simulink model "sampleModel1_pp_1_1"  (R2021b)
settings: Solver=VariableStepAuto  StartTime=0.0  StopTime=10.0  RelTol=1e-3
undefined symbols (not defined in the file or in its folder): DiscIntNeverNeededParam, Newton, Raphson
libraries: simulink x18, slpidlib x4
settings Model: Creator=user  LastModifiedBy=cemery

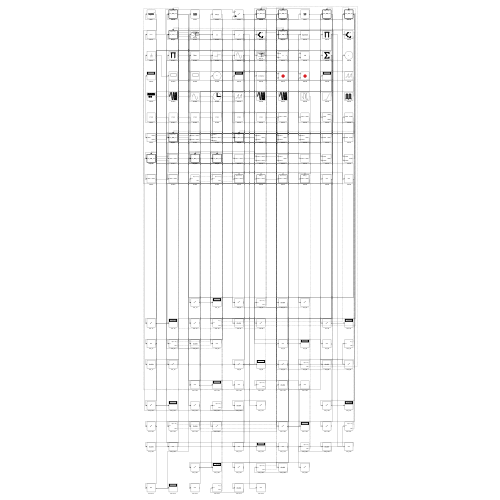
[thumbnail: Simulink's stored preview of the top-level diagram]
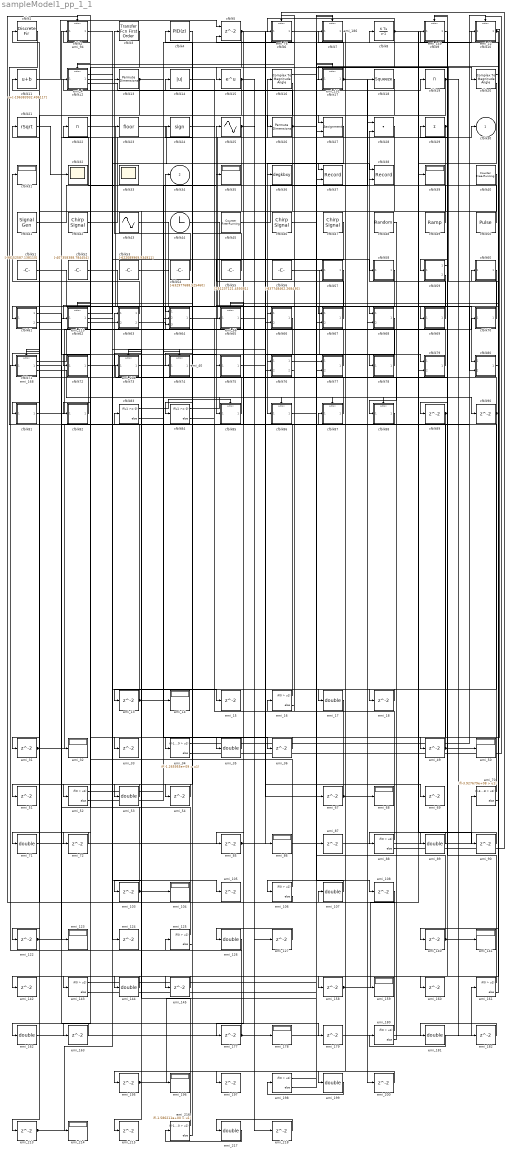
== system sampleModel1_pp_1_1 ==
  cfblk1 : DiscreteFir  SampleTime=1
  cfblk10 : Subsystem  TreatAsAtomicUnit=on
  cfblk11 : Bias  Bias=[-196383932.496117]
  cfblk12 : Subsystem  TreatAsAtomicUnit=on
  cfblk13 : PermuteDimensions
  cfblk14 : Abs
  cfblk15 : Math  SaturateOnIntegerOverflow=on
  cfblk16 : ComplexToMagnitudeAngle
  cfblk17 : Subsystem  TreatAsAtomicUnit=on
  cfblk18 : Squeeze
  cfblk19 : Product  Inputs=*
  cfblk2 : Subsystem  TreatAsAtomicUnit=on
  cfblk20 : ComplexToMagnitudeAngle
  cfblk21 : Sqrt  Operator=rSqrt  AlgorithmType=Newton-Raphson  SaturateOnIntegerOverflow=on
  cfblk22 : Product  Inputs=*
  cfblk23 : Rounding
  cfblk24 : Signum
  cfblk25 : Sin  TimeSource=Use external signal  SampleTime=0
  cfblk26 : PermuteDimensions
  cfblk27 : Assignment  DiagnosticForDimensions=Warning  IndexOptions=Index vector (dialog)  Indices=1  OutputSizes=1
  cfblk28 : DotProduct  InputSameDT=on  OutDataTypeStr=Inherit: Inherit via internal rule
  cfblk29 : Sum  Inputs=+
  cfblk3 : simulink/Discrete/Transfer Fcn First Order  PoleZ=0.95  ICPrevOutput=0.0  DoSatur=off
  cfblk31 : Display
  cfblk32 : Scope
  cfblk33 : Scope
      settings: Floating=on
  cfblk35 : Display
  cfblk36 : ToWorkspace  VariableName=degkbxy  SaveFormat=Timeseries  SampleTime=-1
  cfblk37 : Record  FileSettingsInternal="{\"entries\":[{\"content\":{\"excelSettings\":{\"content\":{},\"type\":\"Streamout.ExcelSettings\"}},\"type\":\"Streamout.FileSettingStorage\",\"uuid\":\"f10d7984-3c8e-4a01-b437-64e6950a7f1c\"}],\"packageUris\":[\"http://schema.mathworks.com/mf0/streamout_blocks/R2020a\"],\"version\":\"1.0\"}"  Layout=[1 1]  SignalsInternal="{\"entries\":[{\"content\":{\"signals\":[{\"content\":{\"blockPath\":[\"sampleModel1_pp_1_1/cfblk37\"],\"channel\":[],\"dimensions\":[1],\"domain\":\"sampleModel1_pp_1_1/cfblk37\",\"lineColor\":\"#77ac30\",\"plots\":[],\"port\":1,\"sid\":[\"\"],\"signalID\":978,\"signalName\":\"cfblk14\"},\"type\":\"RecordBlkView.Signal\",\"uuid\":\"64c2965d-c8c3-42f9-aeb4-1a9e7a6147a8\"},{\"content\":{\"blockPath\":[\"sampleModel1_pp_1_1/cfblk37\"],\"channel\":[],\"dimensions\":[1],\"domain\":\"sampleModel1_pp_1_1/cfblk37\",\"lineColor\":\"#4dbeee\",\"plots\":[],\"port\":2,\"sid\":[\"\"],\"signalID\":982,\"signalName\":\"cfblk16:1\"},\"type\":\"RecordBlkView.Signal\",\"uuid\":\"42395b9b-3004-4283-a0bf-fe2a9eef8989\"}]},\"type\":\"RecordBlkView.InputSignals\",\"uuid\":\"5b0a9ef9-d487-431f-a20f-830121fcf74f\"}],\"packageUris\":[\"http://schema.mathworks.com/mf0/streamout_blocks/R2020a\"],\"version\":\"1.0\"}"  VisualizationBindings="{\"xyplotplugin\":{\"info\":[{\"series\":[],\"subplotID\":1}]}}"  CompatibilityTag=XY
  cfblk38 : Record  FileSettingsInternal="{\"entries\":[{\"content\":{\"excelSettings\":{\"content\":{},\"type\":\"Streamout.ExcelSettings\"}},\"type\":\"Streamout.FileSettingStorage\",\"uuid\":\"de5ebdad-7bfa-474c-9602-9eb7a528d104\"}],\"packageUris\":[\"http://schema.mathworks.com/mf0/streamout_blocks/R2020a\"],\"version\":\"1.0\"}"  Layout=[1 1]  SignalsInternal="{\"entries\":[{\"content\":{\"signals\":[{\"content\":{\"blockPath\":[\"sampleModel1_pp_1_1/cfblk38\"],\"channel\":[],\"dimensions\":[1],\"domain\":\"sampleModel1_pp_1_1/cfblk38\",\"lineColor\":\"#a2142f\",\"plots\":[],\"port\":1,\"sid\":[\"\"],\"signalID\":986,\"signalName\":\"cfblk2\"},\"type\":\"RecordBlkView.Signal\",\"uuid\":\"59823cac-66f4-4fb3-a1c8-ec7d4885dc8b\"},{\"content\":{\"blockPath\":[\"sampleModel1_pp_1_1/cfblk38\"],\"channel\":[],\"dimensions\":[1],\"domain\":\"sampleModel1_pp_1_1/cfblk38\",\"lineColor\":\"#139fff\",\"plots\":[],\"port\":2,\"sid\":[\"\"],\"signalID\":990,\"signalName\":\"cfblk49\"},\"type\":\"RecordBlkView.Signal\",\"uuid\":\"f4fb396b-3304-46b4-a061-728441c3573f\"}]},\"type\":\"RecordBlkView.InputSignals\",\"uuid\":\"8e89f174-1f5e-4363-8739-2fa17bc2ac55\"}],\"packageUris\":[\"http://schema.mathworks.com/mf0/streamout_blocks/R2020a\"],\"version\":\"1.0\"}"  VisualizationBindings="{\"xyplotplugin\":{\"info\":[{\"series\":[],\"subplotID\":1}]}}"  CompatibilityTag=XY
  cfblk39 : Display
  cfblk4 : slpidlib/PID Controller  Controller=PID  Form=Parallel  TimeDomain=Discrete-time  UseExternalTs=off  SampleTime=1  IntegratorMethod=Forward Euler  FilterMethod=Forward Euler  ControllerParametersSource=internal  P=1  I=1  D=0  UseFilter=on  N=100  TunerSelectOption=Transfer Function Based (PID Tuner App)  InitialConditionSource=internal  InitialConditionForIntegrator=0  InitialConditionForFilter=0  DifferentiatorICPrevScaledInput=0  ExternalReset=none  TrackingMode=off  Kt=1  LimitOutput=off  SatLimitsSource=internal  UpperSaturationLimit=inf  LowerSaturationLimit=-inf  LinearizeAsGain=off  AntiWindupMode=none  Kb=1  POutMin=[]  POutMax=[]  IOutMin=[]  IOutMax=[]  DOutMin=[]  DOutMax=[]  NOutMin=[]  NOutMax=[]  SumOutMin=[]  SumOutMax=[]  SaturationOutMin=[]  SaturationOutMax=[]  PParamMin=[]  PParamMax=[]  IParamMin=[]  IParamMax=[]  DParamMin=[]  DParamMax=[]  NParamMin=[]  NParamMax=[]  KbParamMin=[]  KbParamMax=[]  KtParamMin=[]  KtParamMax=[]  KbOutMin=[]  KbOutMax=[]  KtOutMin=[]  KtOutMax=[]  IntegratorOutMin=[]  IntegratorOutMax=[]  FilterOutMin=[]  FilterOutMax=[]  SumI1OutMin=[]  SumI1OutMax=[]  SumI2OutMin=[]  SumI2OutMax=[]  SumI3OutMin=[]  SumI3OutMax=[]  SumI4OutMin=[]  SumI4OutMax=[]  SumDOutMin=[]  SumDOutMax=[]  DifferentiatorOutMin=[]  DifferentiatorOutMax=[]  FilterDiffOutCoefMin=[]  FilterDiffOutCoefMax=[]  ReciprocalOutMin=[]  ReciprocalOutMax=[]  SumDenOutMin=[]  SumDenOutMax=[]  SumNumOutMin=[]  SumNumOutMax=[]  DivideOutMin=[]  DivideOutMax=[]  UdiffTsProdOutMin=[]  UdiffTsProdOutMax=[]  NTsProdOutMin=[]  NTsProdOutMax=[]  UintegralTsProdOutMin=[]  UintegralTsProdOutMax=[]  UngainTsProdOutMin=[]  UngainTsProdOutMax=[]  IntegratorContinuousStateAttributes=''  IntegratorStateMustResolveToSignalObject=off  IntegratorRTWStateStorageClass=Auto  FilterContinuousStateAttributes=''  FilterStateMustResolveToSignalObject=off  FilterRTWStateStorageClass=Auto  ParallelPVariant=InternalParameters  IdealPVariant=Disabled  IVariant=InternalParameters  DVariant=InternalParameters  IntegratorVariant=Discrete  SatVariant=Disabled  AWVariant=Passthrough  PCopyVariant=Disabled  TRVariant=Disabled  FdbkBlocksVariant=Forward  IdealPFdbkVariant=Disabled  SatFdbkVariant=Disabled  DerivativeFilterVariant=ForwardEulerFilter  NVariant=InternalParameters  NCopyVariant=Disabled  FilterICVariant=InternalICsFilter  IntegratorICVariant=InternalICs  ExternalResetVariant=Disabled  TRSumVariant=Passthrough  SumFdbkVariant=Disabled  SumVariant=Sum_PID  TsampFilterVariant=InternalTs  TsampNgainVariant=Passthrough  TsampIntegralVariant=Passthrough  ExternalSaturationOutDataTypeStr=Inherit: Same as second input
  cfblk40 : simulink/Sources/Counter Free-Running  NumBits=[29.000000]  tsamp=-1
  cfblk41 : SignalGenerator  WaveForm=square  Amplitude=[-21494723.199962]
  cfblk42 : simulink/Sources/Chirp Signal  f1=[-261506437.759570]  T=[-777594489.412425]  f2=[560504136.642276]
  cfblk43 : Sin  Amplitude=[-220522326.077493]  Bias=[-516617428.172335]  SampleTime=0
  cfblk44 : Clock
  cfblk45 : simulink/Sources/Counter Free-Running  NumBits=[24.000000]  tsamp=-1
  cfblk46 : simulink/Sources/Chirp Signal  f1=[-807090949.663223]  T=[-736053414.787330]  f2=[884101181.550970]
  cfblk47 : simulink/Sources/Chirp Signal  f1=[912269080.459605]  T=[150417190.156931]  f2=[-880440914.105688]
  cfblk48 : RandomNumber  Mean=[-53044.017326]  Variance=[35315.857122]  Seed=[821194040.000000]  SampleTime=0.1
  cfblk49 : simulink/Sources/Ramp  slope=[-9691.931247]  start=[3.108166]  InitialOutput=[-662019.941075]
  cfblk5 : Delay  ShowEnablePort=on  SampleTime=1
      settings: InputPortMap=u0,e6
  cfblk50 : DiscretePulseGenerator  PulseType=Time based  Amplitude=[298230949.912904]  Period=[73172238.834145]  PulseWidth=5  PhaseDelay=[6.000000]
  cfblk51 : Constant  Value=[-98152587.138110]  SampleTime=1
  cfblk52 : Constant  Value=[-407358388.784454]  SampleTime=1
  cfblk53 : Constant  Value=[-622089969.934911]  SampleTime=1
  cfblk54 : Constant  Value=[-632977688.525460]  SampleTime=1
  cfblk55 : Constant  Value=[251237121.459381]  SampleTime=1
  cfblk56 : Constant  Value=[-837748462.268430]  SampleTime=1
  cfblk57 : Subsystem
  cfblk58 : Subsystem
  cfblk59 : Subsystem
  cfblk6 : Subsystem  TreatAsAtomicUnit=on
  cfblk60 : Subsystem
  cfblk61 : Subsystem
  cfblk62 : Subsystem  TreatAsAtomicUnit=on
  cfblk63 : Subsystem
  cfblk64 : Subsystem
  cfblk65 : Subsystem  TreatAsAtomicUnit=on
  cfblk66 : Subsystem
  cfblk67 : Subsystem
  cfblk68 : Subsystem
  cfblk69 : Subsystem
  cfblk7 : Subsystem  TreatAsAtomicUnit=on
  cfblk70 : Subsystem
  cfblk71 : Subsystem  TreatAsAtomicUnit=on
  cfblk72 : Subsystem
  cfblk73 : Subsystem  TreatAsAtomicUnit=on
  cfblk74 : Subsystem  TreatAsAtomicUnit=on
  cfblk75 : Subsystem
  cfblk76 : Subsystem
  cfblk77 : Subsystem
  cfblk78 : Subsystem
  cfblk79 : Subsystem
  cfblk8 : DiscreteIntegrator  ICPrevOutput=DiscIntNeverNeededParam  ICPrevScaledInput=DiscIntNeverNeededParam
  cfblk80 : Subsystem
  cfblk81 : Subsystem
  cfblk82 : Subsystem
  cfblk83 : If  IfExpression=u1 >= 0  SampleTime=1
  cfblk84 : If  IfExpression=u1 >= 0  SampleTime=1
  cfblk85 : Subsystem  TreatAsAtomicUnit=on
  cfblk86 : Subsystem  TreatAsAtomicUnit=on
  cfblk87 : Subsystem  TreatAsAtomicUnit=on
  cfblk88 : Subsystem  TreatAsAtomicUnit=on
  cfblk89 : Delay  SampleTime=1
  cfblk9 : Subsystem  TreatAsAtomicUnit=on
  cfblk90 : Delay  SampleTime=1
  emi_{13,15,31,33,67,69,85,87,103,105,140,142,158,160,195,197} (16 alike) : Delay
  emi_{14,32,50,68,86,104,123,141,159,178,196,214} (12 alike) : Display
  emi_{16,52,88,106,125,143,161,180,198} (9 alike) : If  IfExpression=0 > u1
  emi_{17,35,53,71,89,107,126,144,162,181,199,217} (12 alike) : DataTypeConversion  OutDataTypeStr=double
  emi_{18,90,108,127,163,182} (6 alike) : Delay  InitialCondition=0
  emi_113 : Subsystem  TreatAsAtomicUnit=on
  emi_{49,51,122,124,177,179,213,215} (8 alike) : Delay  SampleTime=1
  emi_131 : Subsystem  TreatAsAtomicUnit=on
  emi_145 : Delay  InitialCondition=0.026958
  emi_149 : Subsystem  TreatAsAtomicUnit=on
  emi_168 : Subsystem  TreatAsAtomicUnit=on
  emi_186 : Subsystem  TreatAsAtomicUnit=on
  emi_200 : Delay  InitialCondition=0.16419
  emi_204 : Subsystem  TreatAsAtomicUnit=on
  emi_216 : If  IfExpression=-1.586211e+00 > u1
  emi_218 : Delay  InitialCondition=-0.79311
  emi_22 : Subsystem  TreatAsAtomicUnit=on
  emi_34 : If  IfExpression=-1.265955e+09 > u1
  emi_36 : Delay  InitialCondition=-632977688.5255
  emi_4 : Subsystem  TreatAsAtomicUnit=on
  emi_40 : Subsystem  TreatAsAtomicUnit=on
  emi_54 : Delay  InitialCondition=711045611.6918
  emi_58 : Subsystem  TreatAsAtomicUnit=on
  emi_70 : If  IfExpression=-3.927679e+08 > u1
  emi_72 : Delay  InitialCondition=-196383937.6215
  emi_76 : Subsystem  TreatAsAtomicUnit=on
  emi_94 : Subsystem  TreatAsAtomicUnit=on
  cfblk30 : Outport
  cfblk34 : Outport  Port=2
  wires:
  cfblk63/1(cfblk2) -> cfblk31/1
  cfblk67/1(cfblk2) -> cfblk25/1
  cfblk44/1 -> cfblk68/1(cfblk1)
  cfblk21/1 -> cfblk32/1
  cfblk79/1(cfblk2) -> cfblk34/1
  cfblk69/1(cfblk2) -> cfblk28/2
  cfblk72/1(cfblk2) -> cfblk29/1
  cfblk70/1(cfblk2) -> cfblk15/1
  cfblk23/1 -> cfblk86/1(cfblk1)
  cfblk43/1 -> cfblk66/1(cfblk1)
  cfblk77/1(cfblk2) -> cfblk11/1
  cfblk48/1 -> cfblk88/1(cfblk1)
  cfblk53/1 -> cfblk80/1(cfblk1)
  cfblk64/1(cfblk2) -> cfblk30/1
  cfblk68/1(cfblk2) -> cfblk76/1(cfblk1)
  cfblk50/1 -> cfblk22/1
  cfblk78/1(cfblk2) -> cfblk4/1
  cfblk85/1(cfblk2) -> cfblk63/1(cfblk1)
  cfblk52/1 -> cfblk69/1(cfblk1)
  cfblk76/1(cfblk2) -> cfblk77/1(cfblk1)
  cfblk1/1 -> cfblk87/1(cfblk1)
  cfblk56/1 -> cfblk79/1(cfblk1)
  cfblk47/1 -> cfblk85/1(cfblk1)
  cfblk45/1 -> cfblk18/1
  cfblk51/1 -> cfblk80/2(cfblk3)
  cfblk59/2(cfblk3) -> cfblk63/2(cfblk4)
  cfblk81/1(cfblk2) -> cfblk70/1(cfblk1)
  cfblk66/1(cfblk2) -> cfblk84/1
  cfblk86/1(cfblk2) -> cfblk57/1(cfblk1)
  cfblk75/1(cfblk2) -> cfblk8/1
  cfblk42/1 -> cfblk16/1
  cfblk4/1 -> cfblk64/1(cfblk1)
  cfblk22/1 -> cfblk64/2(cfblk3)
  cfblk41/1 -> cfblk3/1
  cfblk20/1 -> cfblk67/1(cfblk1)
  cfblk58/1(cfblk2) -> cfblk61/1(cfblk1)
  cfblk49/1 -> cfblk38/2
  cfblk14/1 -> cfblk37/1
  cfblk80/1(cfblk2) -> cfblk60/1(cfblk1)
  cfblk20/2 -> cfblk79/2(cfblk3)
  cfblk54/1 -> cfblk13/1
  cfblk28/1 -> cfblk68/2(cfblk5)
  cfblk87/1(cfblk2) -> cfblk21/1
  cfblk11/1 -> cfblk5/1
  cfblk57/1(cfblk2) -> cfblk67/2(cfblk4)
  cfblk82/1(cfblk2) -> cfblk1/1
  cfblk61/1(cfblk2) -> cfblk75/1(cfblk1)
  cfblk88/1(cfblk2) -> cfblk83/1
  cfblk60/1(cfblk2) -> cfblk81/1(cfblk1)
  cfblk16/1 -> cfblk37/2
  cfblk76/2(cfblk5) -> cfblk5/2
  cfblk18/1 -> cfblk27/2
  cfblk27/1 -> cfblk36/1
  cfblk3/1 -> cfblk72/1(cfblk1)
  cfblk46/1 -> cfblk77/2(cfblk4)
  cfblk16/2 -> cfblk26/1
  cfblk61/2(cfblk3) -> cfblk23/1
  cfblk63/2(cfblk5) -> cfblk64/3(cfblk4)
  cfblk55/1 -> cfblk24/1
  cfblk40/1 -> cfblk82/1(cfblk1)
  cfblk24/1 -> cfblk66/2(cfblk5)
  cfblk83/1 -> cfblk85/Action
  cfblk83/2 -> cfblk86/Action
  cfblk84/1 -> cfblk87/Action
  cfblk84/2 -> cfblk88/Action
  cfblk59/1(cfblk2) -> cfblk89/1
  cfblk90/1 -> cfblk12/1(emi_1), emi_13/1, emi_18/1
  cfblk12/1(emi_2) -> cfblk58/1(cfblk1)
  cfblk12/2(emi_3) -> cfblk19/1
  emi_13/1 -> emi_4/1(emi_11), emi_14/1
  emi_4/1(emi_12) -> emi_15/1
  emi_16/2 -> cfblk12/Action
  emi_16/1 -> emi_4/Action
  emi_17/1 -> emi_16/1
  emi_18/1 -> emi_17/1
  cfblk13/1 -> cfblk10/1(emi_20), emi_31/1, emi_36/1
  emi_31/1 -> emi_22/1(emi_29), emi_32/1
  emi_22/1(emi_30) -> emi_33/1
  emi_34/2 -> cfblk10/Action
  emi_34/1 -> emi_22/Action
  emi_35/1 -> emi_34/1
  emi_36/1 -> emi_35/1
  cfblk29/1 -> cfblk74/1(emi_38), emi_49/1, emi_54/1
  cfblk74/1(emi_39) -> cfblk14/1
  emi_49/1 -> emi_40/1(emi_47), emi_50/1
  emi_40/1(emi_48) -> emi_51/1
  emi_52/2 -> cfblk74/Action
  emi_52/1 -> emi_40/Action
  emi_53/1 -> emi_52/1
  emi_54/1 -> emi_53/1
  cfblk5/1 -> cfblk65/1(emi_56), emi_67/1, emi_72/1
  cfblk65/1(emi_57) -> cfblk78/1(cfblk1)
  emi_67/1 -> emi_58/1(emi_65), emi_68/1
  emi_58/1(emi_66) -> emi_69/1
  emi_70/2 -> cfblk65/Action
  emi_70/1 -> emi_58/Action
  emi_71/1 -> emi_70/1
  emi_72/1 -> emi_71/1
  cfblk8/1 -> cfblk6/1(emi_74), emi_85/1, emi_90/1
  cfblk6/1(emi_75) -> cfblk20/1
  emi_85/1 -> emi_76/1(emi_83), emi_86/1
  emi_76/1(emi_84) -> emi_87/1
  emi_88/2 -> cfblk6/Action
  emi_88/1 -> emi_76/Action
  emi_89/1 -> emi_88/1
  emi_90/1 -> emi_89/1
  cfblk26/1 -> cfblk2/1(emi_92), emi_103/1, emi_108/1
  cfblk2/1(emi_93) -> cfblk38/1
  emi_103/1 -> emi_94/1(emi_101), emi_104/1
  emi_94/1(emi_102) -> emi_105/1
  emi_106/2 -> cfblk2/Action
  emi_106/1 -> emi_94/Action
  emi_107/1 -> emi_106/1
  emi_108/1 -> emi_107/1
  cfblk15/1 -> cfblk62/1(emi_110), emi_122/1, emi_127/1
  cfblk62/1(emi_111) -> cfblk28/1
  cfblk62/2(emi_112) -> cfblk76/2(cfblk4)
  emi_122/1 -> emi_113/1(emi_120), emi_123/1
  emi_113/1(emi_121) -> emi_124/1
  emi_125/2 -> cfblk62/Action
  emi_125/1 -> emi_113/Action
  emi_126/1 -> emi_125/1
  emi_127/1 -> emi_126/1
  cfblk10/1(emi_21) -> cfblk17/1(emi_129), emi_140/1, emi_145/1
  emi_140/1 -> emi_131/1(emi_138), emi_141/1
  emi_131/1(emi_139) -> emi_142/1
  emi_143/2 -> cfblk17/Action
  emi_143/1 -> emi_131/Action
  emi_144/1 -> emi_143/1
  emi_145/1 -> emi_144/1
  cfblk89/1 -> cfblk9/1(emi_147), emi_158/1, emi_163/1
  cfblk9/1(emi_148) -> cfblk59/1(cfblk1)
  emi_158/1 -> emi_149/1(emi_156), emi_159/1
  emi_149/1(emi_157) -> emi_160/1
  emi_161/2 -> cfblk9/Action
  emi_161/1 -> emi_149/Action
  emi_162/1 -> emi_161/1
  emi_163/1 -> emi_162/1
  cfblk19/1 -> cfblk71/1(emi_165), emi_177/1, emi_182/1
  cfblk71/1(emi_166) -> cfblk39/1
  cfblk71/2(emi_167) -> cfblk90/1
  emi_177/1 -> emi_168/1(emi_175), emi_178/1
  emi_168/1(emi_176) -> emi_179/1
  emi_180/2 -> cfblk71/Action
  emi_180/1 -> emi_168/Action
  emi_181/1 -> emi_180/1
  emi_182/1 -> emi_181/1
  cfblk17/1(emi_130) -> cfblk7/1(emi_184), emi_195/1, emi_200/1
  cfblk7/1(emi_185) -> cfblk27/1
  emi_195/1 -> emi_186/1(emi_193), emi_196/1
  emi_186/1(emi_194) -> emi_197/1
  emi_198/2 -> cfblk7/Action
  emi_198/1 -> emi_186/Action
  emi_199/1 -> emi_198/1
  emi_200/1 -> emi_199/1
  cfblk25/1 -> cfblk73/1(emi_202), emi_213/1, emi_218/1
  cfblk73/1(emi_203) -> cfblk35/1
  emi_213/1 -> emi_204/1(emi_211), emi_214/1
  emi_204/1(emi_212) -> emi_215/1
  emi_216/2 -> cfblk73/Action
  emi_216/1 -> emi_204/Action
  emi_217/1 -> emi_216/1
  emi_218/1 -> emi_217/1

== system sampleModel1_pp_1_1/cfblk10 ==
  emi_20 : Inport
  Action Port : ActionPort  ActionPortLabel=else
  cfblk10 : Trigonometry
  emi_21 : Outport
  wires:
  emi_20/1 -> cfblk10/1
  cfblk10/1 -> emi_21/1

== system sampleModel1_pp_1_1/cfblk12 ==
  emi_1 : Inport
  Action Port : ActionPort  ActionPortLabel=else
  cfblk12 : ComplexToMagnitudeAngle
  emi_2 : Outport
  emi_3 : Outport  Port=2
  wires:
  emi_1/1 -> cfblk12/1
  cfblk12/1 -> emi_2/1
  cfblk12/2 -> emi_3/1

== system sampleModel1_pp_1_1/cfblk17 ==
  emi_129 : Inport
  Action Port : ActionPort  ActionPortLabel=else
  cfblk17 : Sqrt  SaturateOnIntegerOverflow=on
  emi_130 : Outport
  wires:
  emi_129/1 -> cfblk17/1
  cfblk17/1 -> emi_130/1

== system sampleModel1_pp_1_1/cfblk2 ==
  emi_92 : Inport
  Action Port : ActionPort  ActionPortLabel=else
  cfblk2 : simulink/Discrete/Transfer Fcn First Order  PoleZ=0.95  ICPrevOutput=0.0  DoSatur=off
  emi_93 : Outport
  wires:
  emi_92/1 -> cfblk2/1
  cfblk2/1 -> emi_93/1

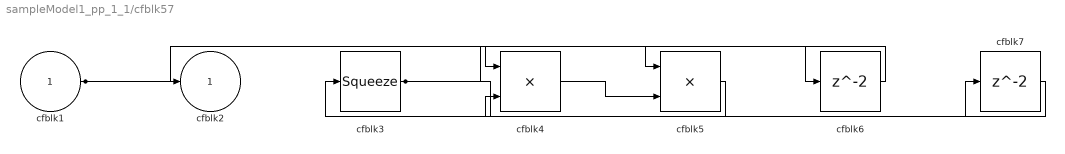
== system sampleModel1_pp_1_1/cfblk57 ==
  cfblk1 : Inport
  cfblk3 : Squeeze
  cfblk4 : Product
  cfblk5 : Product
  cfblk6 : Delay  SampleTime=1
  cfblk7 : Delay  SampleTime=1
  cfblk2 : Outport
  wires:
  cfblk3/1 -> cfblk6/1, cfblk7/1
  cfblk5/1 -> cfblk3/1
  cfblk1/1 -> cfblk4/1, cfblk2/1
  cfblk4/1 -> cfblk5/2
  cfblk6/1 -> cfblk5/1
  cfblk7/1 -> cfblk4/2

== system sampleModel1_pp_1_1/cfblk58 ==
  cfblk1 : Inport
  cfblk3 : DotProduct  InputSameDT=on  OutDataTypeStr=Inherit: Inherit via internal rule
  cfblk2 : Outport
  wires:
  cfblk1/1 -> cfblk3/1, cfblk3/2
  cfblk3/1 -> cfblk2/1

== system sampleModel1_pp_1_1/cfblk59 ==
  cfblk1 : Inport
  cfblk2 : Outport
  cfblk3 : Outport  Port=2
  wires:
  cfblk1/1 -> cfblk2/1, cfblk3/1

== system sampleModel1_pp_1_1/cfblk6 ==
  emi_74 : Inport
  Action Port : ActionPort  ActionPortLabel=else
  cfblk6 : simulink/Discrete/Difference  ICPrevInput=0.0  OutMin=[]  OutMax=[]  OutDataTypeStr=Inherit: Inherit via back propagation  OutDataType=fixdt(1, 16)  OutScaling=2^-10  DoSatur=off
  emi_75 : Outport
  wires:
  emi_74/1 -> cfblk6/1
  cfblk6/1 -> emi_75/1

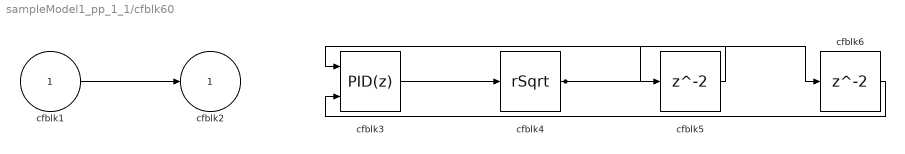
== system sampleModel1_pp_1_1/cfblk60 ==
  cfblk1 : Inport
  cfblk3 : slpidlib/PID Controller (2DOF)  Controller=PID  Form=Parallel  TimeDomain=Discrete-time  UseExternalTs=off  SampleTime=1  IntegratorMethod=Forward Euler  FilterMethod=Forward Euler  ControllerParametersSource=internal  P=1  I=1  D=0  UseFilter=on  N=100  b=1  c=1  TunerSelectOption=Transfer Function Based (PID Tuner App)  InitialConditionSource=internal  InitialConditionForIntegrator=0  InitialConditionForFilter=0  DifferentiatorICPrevScaledInput=0  ExternalReset=none  TrackingMode=off  Kt=1  LimitOutput=off  SatLimitsSource=internal  UpperSaturationLimit=inf  LowerSaturationLimit=-inf  LinearizeAsGain=off  AntiWindupMode=none  Kb=1  POutMin=[]  POutMax=[]  IOutMin=[]  IOutMax=[]  DOutMin=[]  DOutMax=[]  NOutMin=[]  NOutMax=[]  bOutMin=[]  bOutMax=[]  cOutMin=[]  cOutMax=[]  SumOutMin=[]  SumOutMax=[]  SaturationOutMin=[]  SaturationOutMax=[]  PParamMin=[]  PParamMax=[]  IParamMin=[]  IParamMax=[]  DParamMin=[]  DParamMax=[]  NParamMin=[]  NParamMax=[]  bParamMin=[]  bParamMax=[]  cParamMin=[]  cParamMax=[]  KbParamMin=[]  KbParamMax=[]  KtParamMin=[]  KtParamMax=[]  KbOutMin=[]  KbOutMax=[]  KtOutMin=[]  KtOutMax=[]  IntegratorOutMin=[]  IntegratorOutMax=[]  FilterOutMin=[]  FilterOutMax=[]  SumI1OutMin=[]  SumI1OutMax=[]  SumI2OutMin=[]  SumI2OutMax=[]  SumI3OutMin=[]  SumI3OutMax=[]  SumI4OutMin=[]  SumI4OutMax=[]  SumDOutMin=[]  SumDOutMax=[]  Sum1OutMin=[]  Sum1OutMax=[]  Sum2OutMin=[]  Sum2OutMax=[]  Sum3OutMin=[]  Sum3OutMax=[]  DifferentiatorOutMin=[]  DifferentiatorOutMax=[]  FilterDiffOutCoefMin=[]  FilterDiffOutCoefMax=[]  ReciprocalOutMin=[]  ReciprocalOutMax=[]  SumDenOutMin=[]  SumDenOutMax=[]  SumNumOutMin=[]  SumNumOutMax=[]  DivideOutMin=[]  DivideOutMax=[]  UdiffTsProdOutMin=[]  UdiffTsProdOutMax=[]  NTsProdOutMin=[]  NTsProdOutMax=[]  UintegralTsProdOutMin=[]  UintegralTsProdOutMax=[]  UngainTsProdOutMin=[]  UngainTsProdOutMax=[]  IntegratorContinuousStateAttributes=''  IntegratorStateMustResolveToSignalObject=off  IntegratorRTWStateStorageClass=Auto  FilterContinuousStateAttributes=''  FilterStateMustResolveToSignalObject=off  FilterRTWStateStorageClass=Auto  ParallelPVariant=InternalParameters  IdealPVariant=Disabled  IVariant=InternalParameters  DVariant=InternalParameters  bVariant=InternalParameters  cVariant=InternalParameters  IntegratorVariant=Discrete  SatVariant=Disabled  AWVariant=Passthrough  PCopyVariant=Disabled  TRVariant=Disabled  FdbkBlocksVariant=Forward  IdealPFdbkVariant=Disabled  SatFdbkVariant=Disabled  DerivativeFilterVariant=ForwardEulerFilter  NVariant=InternalParameters  NCopyVariant=Disabled  FilterICVariant=InternalICsFilter  IntegratorICVariant=InternalICs  ExternalResetVariant=Disabled  TRSumVariant=Passthrough  SumFdbkVariant=Disabled  SumVariant=Sum_PID  TsampFilterVariant=InternalTs  TsampNgainVariant=Passthrough  TsampIntegralVariant=Passthrough  ExternalSaturationOutDataTypeStr=Inherit: Same as second input
      settings: SourceProductBaseCode=SL
  cfblk4 : Sqrt  Operator=rSqrt  AlgorithmType=Newton-Raphson  SaturateOnIntegerOverflow=on
  cfblk5 : Delay  SampleTime=1
  cfblk6 : Delay  SampleTime=1
  cfblk2 : Outport
  wires:
  cfblk4/1 -> cfblk5/1, cfblk6/1
  cfblk1/1 -> cfblk2/1
  cfblk3/1 -> cfblk4/1
  cfblk5/1 -> cfblk3/1
  cfblk6/1 -> cfblk3/2

== system sampleModel1_pp_1_1/cfblk61 ==
  cfblk1 : Inport
  cfblk2 : Outport
  cfblk3 : Outport  Port=2
  wires:
  cfblk1/1 -> cfblk3/1, cfblk2/1

== system sampleModel1_pp_1_1/cfblk62 ==
  emi_110 : Inport
  Action Port : ActionPort  ActionPortLabel=else
  cfblk62 : Subsystem
  emi_111 : Outport
  emi_112 : Outport  Port=2
  wires:
  emi_110/1 -> cfblk62/1(cfblk1)
  cfblk62/1(cfblk2) -> emi_111/1
  cfblk62/2(cfblk4) -> emi_112/1

== system sampleModel1_pp_1_1/cfblk63 ==
  cfblk1 : Inport
  cfblk4 : Inport  Port=2
  cfblk3 : DiscreteFir  SampleTime=1
  cfblk2 : Outport
  cfblk5 : Outport  Port=2
  wires:
  cfblk4/1 -> cfblk3/1
  cfblk3/1 -> cfblk2/1
  cfblk1/1 -> cfblk5/1

== system sampleModel1_pp_1_1/cfblk64 ==
  cfblk1 : Inport
  cfblk3 : Inport  Port=2
  cfblk4 : Inport  Port=3
  cfblk2 : Outport
  wires:
  cfblk4/1 -> cfblk2/1

== system sampleModel1_pp_1_1/cfblk65 ==
  emi_56 : Inport
  Action Port : ActionPort  ActionPortLabel=else
  cfblk65 : Subsystem
  emi_57 : Outport
  wires:
  emi_56/1 -> cfblk65/1(cfblk1)
  cfblk65/1(cfblk2) -> emi_57/1

== system sampleModel1_pp_1_1/cfblk66 ==
  cfblk1 : Inport
  cfblk5 : Inport  Port=2
  cfblk3 : simulink/Discrete/Transfer Fcn Real Zero  ZeroZ=0.75  ICPrevInput=0.0  DoSatur=off
      settings: SourceProductBaseCode=SL
  cfblk4 : Sum
  cfblk2 : Outport
  wires:
  cfblk5/1 -> cfblk4/1
  cfblk1/1 -> cfblk3/1
  cfblk4/1 -> cfblk2/1
  cfblk3/1 -> cfblk4/2

== system sampleModel1_pp_1_1/cfblk67 ==
  cfblk1 : Inport
  cfblk4 : Inport  Port=2
  cfblk3 : simulink/Discrete/Transfer Fcn Lead or Lag  PoleZ=0.95  ZeroZ=0.75  ICPrevOutput=0.0  ICPrevInput=0.0  DoSatur=off
      settings: SourceProductBaseCode=SL
  cfblk2 : Outport
  wires:
  cfblk1/1 -> cfblk3/1
  cfblk4/1 -> cfblk2/1

== system sampleModel1_pp_1_1/cfblk68 ==
  cfblk1 : Inport
  cfblk5 : Inport  Port=2
  cfblk3 : simulink/Math Operations/MinMax Running Resettable  Function=min  vinit=0.0
  cfblk4 : Constant  Value=[650627590.804091]  SampleTime=1
  cfblk2 : Outport
  wires:
  cfblk1/1 -> cfblk2/1
  cfblk5/1 -> cfblk3/1
  cfblk4/1 -> cfblk3/2

== system sampleModel1_pp_1_1/cfblk69 ==
  cfblk1 : Inport
  cfblk3 : Rounding
  cfblk4 : Reshape
  cfblk2 : Outport
  wires:
  cfblk3/1 -> cfblk2/1
  cfblk4/1 -> cfblk3/1
  cfblk1/1 -> cfblk4/1

== system sampleModel1_pp_1_1/cfblk7 ==
  emi_184 : Inport
  Action Port : ActionPort  ActionPortLabel=else
  cfblk7 : simulink/Discrete/Difference  ICPrevInput=0.0  OutMin=[]  OutMax=[]  OutDataTypeStr=Inherit: Inherit via back propagation  OutDataType=fixdt(1, 16)  OutScaling=2^-10  DoSatur=off
  emi_185 : Outport
  wires:
  emi_184/1 -> cfblk7/1
  cfblk7/1 -> emi_185/1

== system sampleModel1_pp_1_1/cfblk70 ==
  cfblk1 : Inport
  cfblk3 : DiscreteFilter  SampleTime=1
  cfblk4 : UnaryMinus
  cfblk2 : Outport
  wires:
  cfblk1/1 -> cfblk4/1
  cfblk4/1 -> cfblk3/1
  cfblk3/1 -> cfblk2/1

== system sampleModel1_pp_1_1/cfblk71 ==
  emi_165 : Inport
  Action Port : ActionPort  ActionPortLabel=else
  cfblk71 : Subsystem
  emi_166 : Outport
  emi_167 : Outport  Port=2
  wires:
  emi_165/1 -> cfblk71/1(cfblk1)
  cfblk71/1(cfblk2) -> emi_166/1
  cfblk71/2(cfblk5) -> emi_167/1

== system sampleModel1_pp_1_1/cfblk72 ==
  cfblk1 : Inport
  cfblk3 : DiscreteStateSpace
  cfblk4 : ComplexToMagnitudeAngle
  cfblk5 : Constant  Value=[711045611.691823]  SampleTime=1
  cfblk2 : Outport
  wires:
  cfblk1/1 -> cfblk3/1
  cfblk4/1 -> cfblk2/1
  cfblk5/1 -> cfblk4/1

== system sampleModel1_pp_1_1/cfblk73 ==
  emi_202 : Inport
  Action Port : ActionPort  ActionPortLabel=else
  cfblk73 : Subsystem
  emi_203 : Outport
  wires:
  emi_202/1 -> cfblk73/1(cfblk1)
  cfblk73/1(cfblk2) -> emi_203/1

== system sampleModel1_pp_1_1/cfblk74 ==
  emi_38 : Inport
  Action Port : ActionPort  ActionPortLabel=else
  cfblk74 : Subsystem
  emi_39 : Outport
  wires:
  emi_38/1 -> cfblk74/1(cfblk1)
  cfblk74/1(cfblk2) -> emi_39/1

== system sampleModel1_pp_1_1/cfblk75 ==
  cfblk1 : Inport
  cfblk3 : DiscreteStateSpace
  cfblk4 : Reshape
  cfblk5 : Delay  SampleTime=1
  cfblk2 : Outport
  wires:
  cfblk1/1 -> cfblk2/1
  cfblk3/1 -> cfblk4/1
  cfblk4/1 -> cfblk5/1
  cfblk5/1 -> cfblk3/1

== system sampleModel1_pp_1_1/cfblk76 ==
  cfblk1 : Inport
  cfblk4 : Inport  Port=2
  cfblk3 : Assignment  DiagnosticForDimensions=Warning  IndexOptions=Index vector (dialog)  Indices=1  OutputSizes=1
  cfblk2 : Outport
  cfblk5 : Outport  Port=2
  wires:
  cfblk4/1 -> cfblk3/1
  cfblk1/1 -> cfblk3/2
  cfblk3/1 -> cfblk2/1, cfblk5/1

== system sampleModel1_pp_1_1/cfblk77 ==
  cfblk1 : Inport
  cfblk4 : Inport  Port=2
  cfblk3 : Product
  cfblk2 : Outport
  wires:
  cfblk4/1 -> cfblk3/1
  cfblk1/1 -> cfblk3/2
  cfblk3/1 -> cfblk2/1

== system sampleModel1_pp_1_1/cfblk78 ==
  cfblk1 : Inport
  cfblk3 : simulink/Discrete/Transfer Fcn Lead or Lag  PoleZ=0.95  ZeroZ=0.75  ICPrevOutput=0.0  ICPrevInput=0.0  DoSatur=off
      settings: SourceProductBaseCode=SL
  cfblk4 : Math  Operator=mod  SaturateOnIntegerOverflow=on
  cfblk5 : Constant  Value=[350664131.493999]  SampleTime=1
  cfblk2 : Outport
  wires:
  cfblk4/1 -> cfblk3/1
  cfblk1/1 -> cfblk4/1
  cfblk3/1 -> cfblk2/1
  cfblk5/1 -> cfblk4/2

== system sampleModel1_pp_1_1/cfblk79 ==
  cfblk1 : Inport
  cfblk3 : Inport  Port=2
  cfblk2 : Outport
  wires:
  cfblk1/1 -> cfblk2/1

== system sampleModel1_pp_1_1/cfblk80 ==
  cfblk1 : Inport
  cfblk3 : Inport  Port=2
  cfblk2 : Outport
  wires:
  cfblk1/1 -> cfblk2/1

== system sampleModel1_pp_1_1/cfblk81 ==
  cfblk1 : Inport
  cfblk3 : simulink/Discrete/Tapped Delay  vinit=0.0  samptime=-1  NumDelays=1  DelayOrder=Oldest  includeCurrent=off
  cfblk4 : DotProduct  InputSameDT=on  OutDataTypeStr=Inherit: Inherit via internal rule
  cfblk2 : Outport
  wires:
  cfblk4/1 -> cfblk2/1
  cfblk1/1 -> cfblk3/1
  cfblk3/1 -> cfblk4/1, cfblk4/2

== system sampleModel1_pp_1_1/cfblk82 ==
  cfblk1 : Inport
  cfblk3 : Constant  Value=[358033508.186404]  SampleTime=1
  cfblk4 : Constant  Value=[890348226.218803]  SampleTime=1
  cfblk2 : Outport
  wires:
  cfblk1/1 -> cfblk2/1

== system sampleModel1_pp_1_1/cfblk85 ==
  cfblk1 : Inport
  Action Port : ActionPort  ActionPortLabel=if(u1 >= 0)
  cfblk3 : simulink/Math Operations/Slider Gain  gain=1  low=0  high=2
  cfblk4 : Constant  Value=[-299563973.117790]  SampleTime=1
  cfblk2 : Outport
  wires:
  cfblk4/1 -> cfblk2/1
  cfblk1/1 -> cfblk3/1

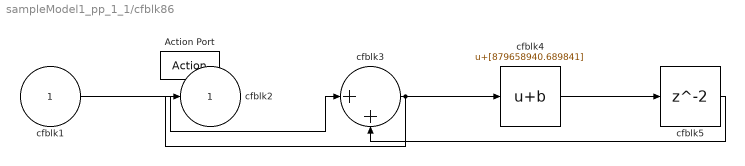
== system sampleModel1_pp_1_1/cfblk86 ==
  cfblk1 : Inport
  Action Port : ActionPort  ActionPortLabel=else
  cfblk3 : Sum  Inputs=|++
  cfblk4 : Bias  Bias=[879658940.689841]
  cfblk5 : Delay
  cfblk2 : Outport
  wires:
  cfblk1/1 -> cfblk3/1
  cfblk3/1 -> cfblk4/1, cfblk2/1
  cfblk4/1 -> cfblk5/1
  cfblk5/1 -> cfblk3/2

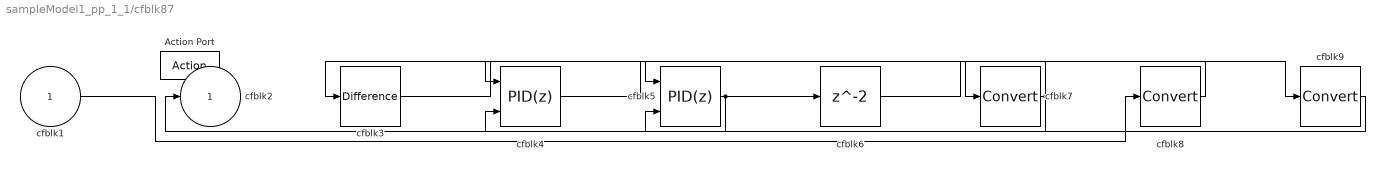
== system sampleModel1_pp_1_1/cfblk87 ==
  cfblk1 : Inport
  Action Port : ActionPort  ActionPortLabel=if(u1 >= 0)
  cfblk3 : simulink/Discrete/Difference  ICPrevInput=0.0  OutMin=[]  OutMax=[]  OutDataTypeStr=Inherit: Inherit via back propagation  OutDataType=fixdt(1, 16)  OutScaling=2^-10  DoSatur=off
  cfblk4 : slpidlib/PID Controller (2DOF)  Controller=PID  Form=Parallel  TimeDomain=Discrete-time  UseExternalTs=off  SampleTime=-1  IntegratorMethod=Forward Euler  FilterMethod=Forward Euler  ControllerParametersSource=internal  P=1  I=1  D=0  UseFilter=on  N=100  b=1  c=1  TunerSelectOption=Transfer Function Based (PID Tuner App)  InitialConditionSource=internal  InitialConditionForIntegrator=0  InitialConditionForFilter=0  DifferentiatorICPrevScaledInput=0  ExternalReset=none  TrackingMode=off  Kt=1  LimitOutput=off  SatLimitsSource=internal  UpperSaturationLimit=inf  LowerSaturationLimit=-inf  LinearizeAsGain=off  AntiWindupMode=none  Kb=1  POutMin=[]  POutMax=[]  IOutMin=[]  IOutMax=[]  DOutMin=[]  DOutMax=[]  NOutMin=[]  NOutMax=[]  bOutMin=[]  bOutMax=[]  cOutMin=[]  cOutMax=[]  SumOutMin=[]  SumOutMax=[]  SaturationOutMin=[]  SaturationOutMax=[]  PParamMin=[]  PParamMax=[]  IParamMin=[]  IParamMax=[]  DParamMin=[]  DParamMax=[]  NParamMin=[]  NParamMax=[]  bParamMin=[]  bParamMax=[]  cParamMin=[]  cParamMax=[]  KbParamMin=[]  KbParamMax=[]  KtParamMin=[]  KtParamMax=[]  KbOutMin=[]  KbOutMax=[]  KtOutMin=[]  KtOutMax=[]  IntegratorOutMin=[]  IntegratorOutMax=[]  FilterOutMin=[]  FilterOutMax=[]  SumI1OutMin=[]  SumI1OutMax=[]  SumI2OutMin=[]  SumI2OutMax=[]  SumI3OutMin=[]  SumI3OutMax=[]  SumI4OutMin=[]  SumI4OutMax=[]  SumDOutMin=[]  SumDOutMax=[]  Sum1OutMin=[]  Sum1OutMax=[]  Sum2OutMin=[]  Sum2OutMax=[]  Sum3OutMin=[]  Sum3OutMax=[]  DifferentiatorOutMin=[]  DifferentiatorOutMax=[]  FilterDiffOutCoefMin=[]  FilterDiffOutCoefMax=[]  ReciprocalOutMin=[]  ReciprocalOutMax=[]  SumDenOutMin=[]  SumDenOutMax=[]  SumNumOutMin=[]  SumNumOutMax=[]  DivideOutMin=[]  DivideOutMax=[]  UdiffTsProdOutMin=[]  UdiffTsProdOutMax=[]  NTsProdOutMin=[]  NTsProdOutMax=[]  UintegralTsProdOutMin=[]  UintegralTsProdOutMax=[]  UngainTsProdOutMin=[]  UngainTsProdOutMax=[]  IntegratorContinuousStateAttributes=''  IntegratorStateMustResolveToSignalObject=off  IntegratorRTWStateStorageClass=Auto  FilterContinuousStateAttributes=''  FilterStateMustResolveToSignalObject=off  FilterRTWStateStorageClass=Auto  ParallelPVariant=InternalParameters  IdealPVariant=Disabled  IVariant=InternalParameters  DVariant=InternalParameters  bVariant=InternalParameters  cVariant=InternalParameters  IntegratorVariant=Discrete  SatVariant=Disabled  AWVariant=Passthrough  PCopyVariant=Disabled  TRVariant=Disabled  FdbkBlocksVariant=Forward  IdealPFdbkVariant=Disabled  SatFdbkVariant=Disabled  DerivativeFilterVariant=ForwardEulerFilter  NVariant=InternalParameters  NCopyVariant=Disabled  FilterICVariant=InternalICsFilter  IntegratorICVariant=InternalICs  ExternalResetVariant=Disabled  TRSumVariant=Passthrough  SumFdbkVariant=Disabled  SumVariant=Sum_PID  TsampFilterVariant=InternalTs  TsampNgainVariant=Passthrough  TsampIntegralVariant=Passthrough  ExternalSaturationOutDataTypeStr=Inherit: Same as second input
      settings: SourceProductBaseCode=SL
  cfblk5 : slpidlib/PID Controller (2DOF)  Controller=PID  Form=Parallel  TimeDomain=Discrete-time  UseExternalTs=off  SampleTime=-1  IntegratorMethod=Forward Euler  FilterMethod=Forward Euler  ControllerParametersSource=internal  P=1  I=1  D=0  UseFilter=on  N=100  b=1  c=1  TunerSelectOption=Transfer Function Based (PID Tuner App)  InitialConditionSource=internal  InitialConditionForIntegrator=0  InitialConditionForFilter=0  DifferentiatorICPrevScaledInput=0  ExternalReset=none  TrackingMode=off  Kt=1  LimitOutput=off  SatLimitsSource=internal  UpperSaturationLimit=inf  LowerSaturationLimit=-inf  LinearizeAsGain=off  AntiWindupMode=none  Kb=1  POutMin=[]  POutMax=[]  IOutMin=[]  IOutMax=[]  DOutMin=[]  DOutMax=[]  NOutMin=[]  NOutMax=[]  bOutMin=[]  bOutMax=[]  cOutMin=[]  cOutMax=[]  SumOutMin=[]  SumOutMax=[]  SaturationOutMin=[]  SaturationOutMax=[]  PParamMin=[]  PParamMax=[]  IParamMin=[]  IParamMax=[]  DParamMin=[]  DParamMax=[]  NParamMin=[]  NParamMax=[]  bParamMin=[]  bParamMax=[]  cParamMin=[]  cParamMax=[]  KbParamMin=[]  KbParamMax=[]  KtParamMin=[]  KtParamMax=[]  KbOutMin=[]  KbOutMax=[]  KtOutMin=[]  KtOutMax=[]  IntegratorOutMin=[]  IntegratorOutMax=[]  FilterOutMin=[]  FilterOutMax=[]  SumI1OutMin=[]  SumI1OutMax=[]  SumI2OutMin=[]  SumI2OutMax=[]  SumI3OutMin=[]  SumI3OutMax=[]  SumI4OutMin=[]  SumI4OutMax=[]  SumDOutMin=[]  SumDOutMax=[]  Sum1OutMin=[]  Sum1OutMax=[]  Sum2OutMin=[]  Sum2OutMax=[]  Sum3OutMin=[]  Sum3OutMax=[]  DifferentiatorOutMin=[]  DifferentiatorOutMax=[]  FilterDiffOutCoefMin=[]  FilterDiffOutCoefMax=[]  ReciprocalOutMin=[]  ReciprocalOutMax=[]  SumDenOutMin=[]  SumDenOutMax=[]  SumNumOutMin=[]  SumNumOutMax=[]  DivideOutMin=[]  DivideOutMax=[]  UdiffTsProdOutMin=[]  UdiffTsProdOutMax=[]  NTsProdOutMin=[]  NTsProdOutMax=[]  UintegralTsProdOutMin=[]  UintegralTsProdOutMax=[]  UngainTsProdOutMin=[]  UngainTsProdOutMax=[]  IntegratorContinuousStateAttributes=''  IntegratorStateMustResolveToSignalObject=off  IntegratorRTWStateStorageClass=Auto  FilterContinuousStateAttributes=''  FilterStateMustResolveToSignalObject=off  FilterRTWStateStorageClass=Auto  ParallelPVariant=InternalParameters  IdealPVariant=Disabled  IVariant=InternalParameters  DVariant=InternalParameters  bVariant=InternalParameters  cVariant=InternalParameters  IntegratorVariant=Discrete  SatVariant=Disabled  AWVariant=Passthrough  PCopyVariant=Disabled  TRVariant=Disabled  FdbkBlocksVariant=Forward  IdealPFdbkVariant=Disabled  SatFdbkVariant=Disabled  DerivativeFilterVariant=ForwardEulerFilter  NVariant=InternalParameters  NCopyVariant=Disabled  FilterICVariant=InternalICsFilter  IntegratorICVariant=InternalICs  ExternalResetVariant=Disabled  TRSumVariant=Passthrough  SumFdbkVariant=Disabled  SumVariant=Sum_PID  TsampFilterVariant=InternalTs  TsampNgainVariant=Passthrough  TsampIntegralVariant=Passthrough  ExternalSaturationOutDataTypeStr=Inherit: Same as second input
      settings: SourceProductBaseCode=SL
  cfblk6 : Delay
  cfblk7 : DataTypeConversion
  cfblk8 : DataTypeConversion
  cfblk9 : DataTypeConversion
  cfblk2 : Outport
  wires:
  cfblk3/1 -> cfblk5/1
  cfblk4/1 -> cfblk7/1
  cfblk5/1 -> cfblk2/1, cfblk6/1
  cfblk7/1 -> cfblk3/1, cfblk5/2
  cfblk1/1 -> cfblk8/1
  cfblk8/1 -> cfblk4/1
  cfblk6/1 -> cfblk9/1
  cfblk9/1 -> cfblk4/2

== system sampleModel1_pp_1_1/cfblk88 ==
  cfblk1 : Inport
  Action Port : ActionPort  ActionPortLabel=else
  cfblk3 : Sin  TimeSource=Use external signal  SampleTime=0
  cfblk4 : Constant  Value=[40104934.780774]  SampleTime=1
  cfblk2 : Outport
  wires:
  cfblk3/1 -> cfblk2/1
  cfblk1/1 -> cfblk3/1

== system sampleModel1_pp_1_1/cfblk9 ==
  emi_147 : Inport
  Action Port : ActionPort  ActionPortLabel=else
  cfblk9 : simulink/Discrete/Transfer Fcn First Order  PoleZ=0.95  ICPrevOutput=0.0  DoSatur=off
  emi_148 : Outport
  wires:
  emi_147/1 -> cfblk9/1
  cfblk9/1 -> emi_148/1

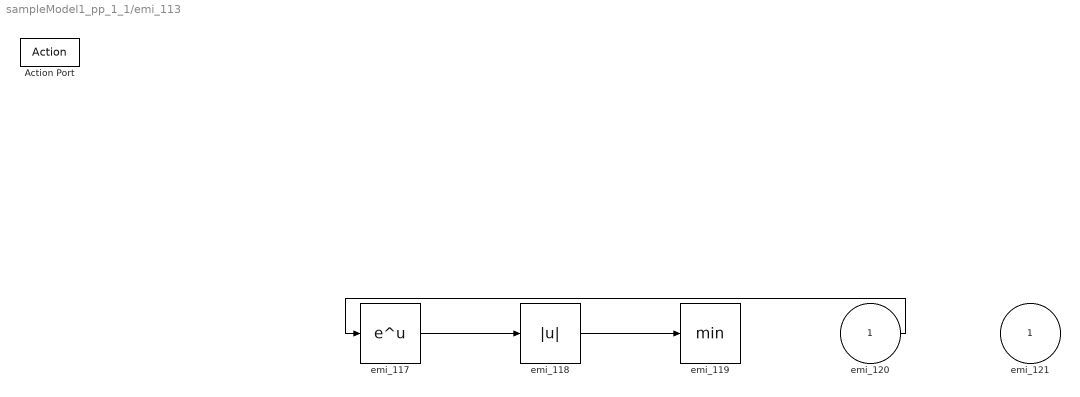
== system sampleModel1_pp_1_1/emi_113 ==
  emi_120 : Inport
  Action Port : ActionPort  ActionPortLabel=if(0 > u1)
  emi_117 : Math  SaturateOnIntegerOverflow=on
  emi_118 : Abs
  emi_119 : MinMax
  emi_121 : Outport
  wires:
  emi_120/1 -> emi_117/1
  emi_117/1 -> emi_118/1
  emi_118/1 -> emi_119/1

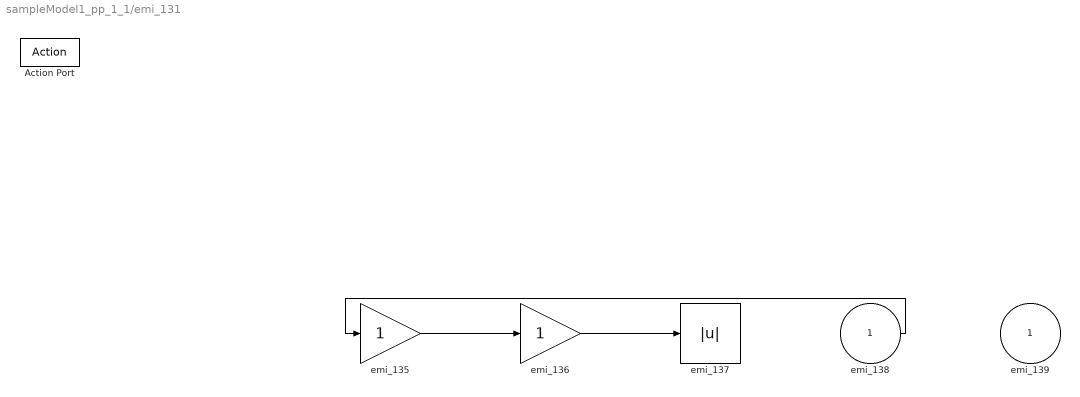
== system sampleModel1_pp_1_1/emi_131 ==
  emi_138 : Inport
  Action Port : ActionPort  ActionPortLabel=if(0 > u1)
  emi_135 : Gain
  emi_136 : Gain
  emi_137 : Abs
  emi_139 : Outport
  wires:
  emi_138/1 -> emi_135/1
  emi_135/1 -> emi_136/1
  emi_136/1 -> emi_137/1

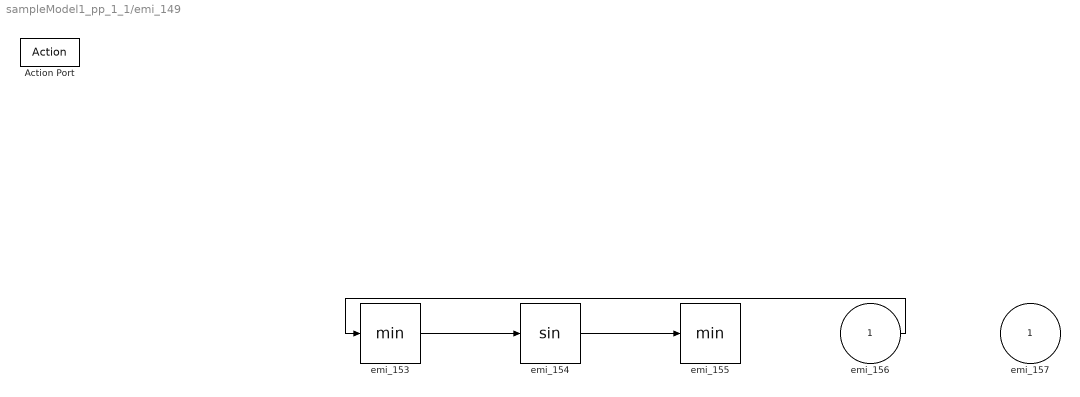
== system sampleModel1_pp_1_1/emi_149 ==
  emi_156 : Inport
  Action Port : ActionPort  ActionPortLabel=if(0 > u1)
  emi_153 : MinMax
  emi_154 : Trigonometry
  emi_155 : MinMax
  emi_157 : Outport
  wires:
  emi_156/1 -> emi_153/1
  emi_153/1 -> emi_154/1
  emi_154/1 -> emi_155/1

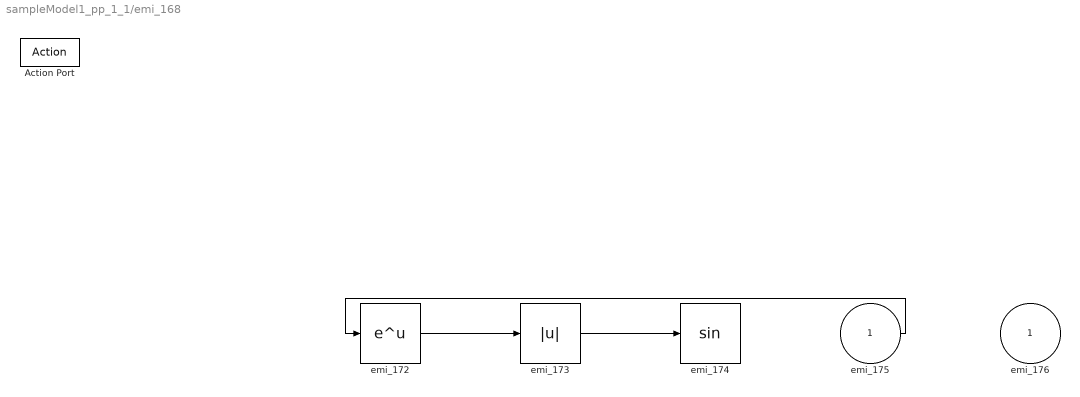
== system sampleModel1_pp_1_1/emi_168 ==
  emi_175 : Inport
  Action Port : ActionPort  ActionPortLabel=if(0 > u1)
  emi_172 : Math  SaturateOnIntegerOverflow=on
  emi_173 : Abs
  emi_174 : Trigonometry
  emi_176 : Outport
  wires:
  emi_175/1 -> emi_172/1
  emi_172/1 -> emi_173/1
  emi_173/1 -> emi_174/1

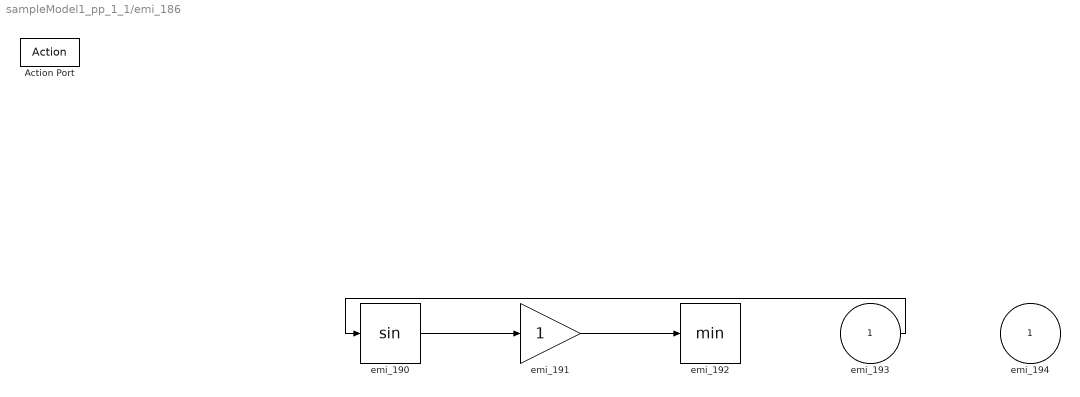
== system sampleModel1_pp_1_1/emi_186 ==
  emi_193 : Inport
  Action Port : ActionPort  ActionPortLabel=if(0 > u1)
  emi_190 : Trigonometry
  emi_191 : Gain
  emi_192 : MinMax
  emi_194 : Outport
  wires:
  emi_193/1 -> emi_190/1
  emi_190/1 -> emi_191/1
  emi_191/1 -> emi_192/1

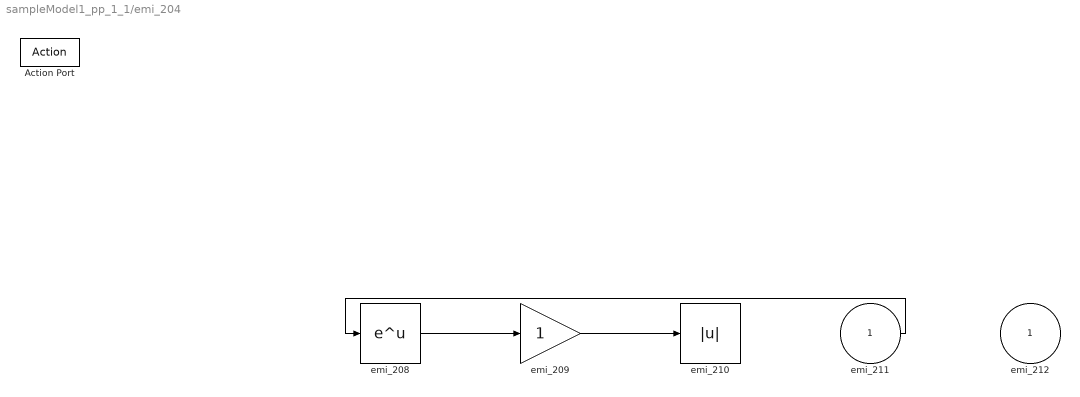
== system sampleModel1_pp_1_1/emi_204 ==
  emi_211 : Inport
  Action Port : ActionPort  ActionPortLabel=if(-1.586211e+00 > u1)
  emi_208 : Math  SaturateOnIntegerOverflow=on
  emi_209 : Gain
  emi_210 : Abs
  emi_212 : Outport
  wires:
  emi_211/1 -> emi_208/1
  emi_208/1 -> emi_209/1
  emi_209/1 -> emi_210/1

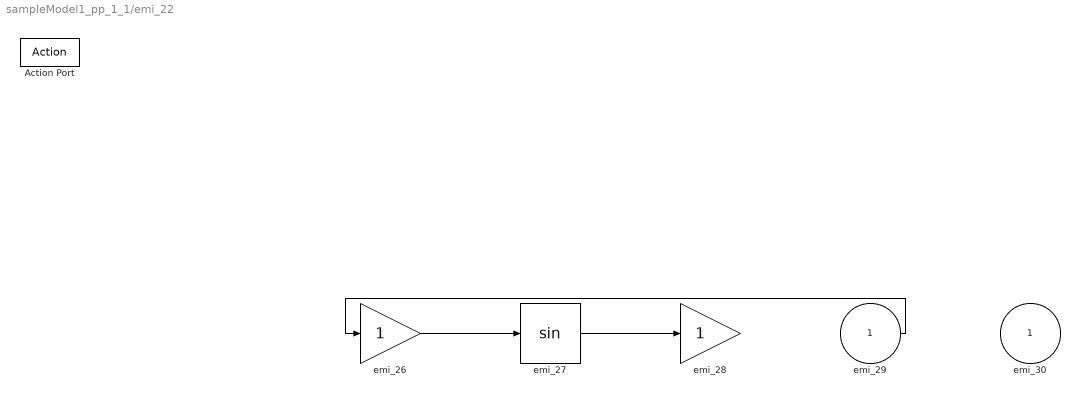
== system sampleModel1_pp_1_1/emi_22 ==
  emi_29 : Inport
  Action Port : ActionPort  ActionPortLabel=if(-1.265955e+09 > u1)
  emi_26 : Gain
  emi_27 : Trigonometry
  emi_28 : Gain
  emi_30 : Outport
  wires:
  emi_29/1 -> emi_26/1
  emi_26/1 -> emi_27/1
  emi_27/1 -> emi_28/1

== system sampleModel1_pp_1_1/emi_4 ==
  emi_11 : Inport
  Action Port : ActionPort  ActionPortLabel=if(0 > u1)
  emi_10 : Math  SaturateOnIntegerOverflow=on
  emi_8 : Trigonometry
  emi_9 : Math  SaturateOnIntegerOverflow=on
  emi_12 : Outport
  wires:
  emi_11/1 -> emi_8/1
  emi_8/1 -> emi_9/1
  emi_9/1 -> emi_10/1

== system sampleModel1_pp_1_1/emi_40 ==
  emi_47 : Inport
  Action Port : ActionPort  ActionPortLabel=if(0 > u1)
  emi_44 : MinMax
  emi_45 : Trigonometry
  emi_46 : Gain
  emi_48 : Outport
  wires:
  emi_47/1 -> emi_44/1
  emi_44/1 -> emi_45/1
  emi_45/1 -> emi_46/1

== system sampleModel1_pp_1_1/emi_58 ==
  emi_65 : Inport
  Action Port : ActionPort  ActionPortLabel=if(-3.927679e+08 > u1)
  emi_62 : MinMax
  emi_63 : Abs
  emi_64 : Math  SaturateOnIntegerOverflow=on
  emi_66 : Outport
  wires:
  emi_65/1 -> emi_62/1
  emi_62/1 -> emi_63/1
  emi_63/1 -> emi_64/1

== system sampleModel1_pp_1_1/emi_76 ==
  emi_83 : Inport
  Action Port : ActionPort  ActionPortLabel=if(0 > u1)
  emi_80 : Math  SaturateOnIntegerOverflow=on
  emi_81 : MinMax
  emi_82 : Gain
  emi_84 : Outport
  wires:
  emi_83/1 -> emi_80/1
  emi_80/1 -> emi_81/1
  emi_81/1 -> emi_82/1

== system sampleModel1_pp_1_1/emi_94 ==
  emi_101 : Inport
  Action Port : ActionPort  ActionPortLabel=if(0 > u1)
  emi_100 : Math  SaturateOnIntegerOverflow=on
  emi_98 : Trigonometry
  emi_99 : Gain
  emi_102 : Outport
  wires:
  emi_101/1 -> emi_98/1
  emi_98/1 -> emi_99/1
  emi_99/1 -> emi_100/1

== system sampleModel1_pp_1_1/cfblk62/cfblk62 ==
  cfblk1 : Inport
  cfblk3 : Product
  cfblk2 : Outport
  cfblk4 : Outport  Port=2
  wires:
  cfblk3/1 -> cfblk4/1
  cfblk1/1 -> cfblk3/2, cfblk3/1, cfblk2/1

== system sampleModel1_pp_1_1/cfblk65/cfblk65 ==
  cfblk1 : Inport
  cfblk3 : Delay  SampleTime=1
  cfblk4 : Constant  Value=[488148520.734925]  SampleTime=1
  cfblk2 : Outport
  wires:
  cfblk1/1 -> cfblk3/1
  cfblk4/1 -> cfblk2/1

== system sampleModel1_pp_1_1/cfblk71/cfblk71 ==
  cfblk1 : Inport
  cfblk3 : Product  Inputs=*
  cfblk4 : Rounding
  cfblk6 : Delay  SampleTime=1
  cfblk2 : Outport
  cfblk5 : Outport  Port=2
  wires:
  cfblk6/1 -> cfblk3/1
  cfblk4/1 -> cfblk6/1, cfblk5/1
  cfblk1/1 -> cfblk2/1
  cfblk3/1 -> cfblk4/1

== system sampleModel1_pp_1_1/cfblk73/cfblk73 ==
  cfblk1 : Inport
  cfblk3 : Gain  Gain=[234181768.786447]
  cfblk2 : Outport
  wires:
  cfblk1/1 -> cfblk3/1
  cfblk3/1 -> cfblk2/1

== system sampleModel1_pp_1_1/cfblk74/cfblk74 ==
  cfblk1 : Inport
  cfblk3 : UnitDelay  HasFrameUpgradeWarning=on
  cfblk4 : Sum  Inputs=|++
  cfblk2 : Outport
  wires:
  cfblk3/1 -> cfblk2/1
  cfblk4/1 -> cfblk3/1
  cfblk1/1 -> cfblk4/2, cfblk4/1
